simulink model "bolide_modele_simul2"  (R2023b)
settings: Solver=VariableStepAuto  StartTime=0.0  StopTime=5.0  RelTol=1e-3
model workspace (MATLAB code in the model file):
  | %% True Parameters
  | % Masses
  | mw=0.1;
  | mb=1;
  | M=1.2;
  | 
  | % Distances
  | rho=0.07;
  | l=0.02;
  | d=0.015; % distance A-C
  | 
  | % Electriques
  | L=0.05;
  | R=1e6;
  | % r;
  | 
  | % Couples
  | k=2.63e4;
  | % alpha=34.6;
  | % beta=2.06e5;
  | 
  | % Moments inertie
  | Iwy=2.45e-4;
  | Ipsi=1.53e-2;
  | 
  | % Utilitaire
  | beta = (M + 2*Iwy/rho^2);
  | gamma = Ipsi + mb*d^2;
  | 
  | %% Nominal Equilibrium Point
  | Ubar = 12;
  | Urbar = Ubar/2;
  | Ulbar = Ubar/2;
  | 
  | ubar = rho/2/k*Ubar; % m/s
  | psibar = 0;
  | vbar = 0;
  | irbar = 0;
  | ilbar = 0;
  | 
  | statebar = [ubar; psibar; vbar; irbar; ilbar];
settings Model: Creator=Jules  LastModifiedBy=Jules

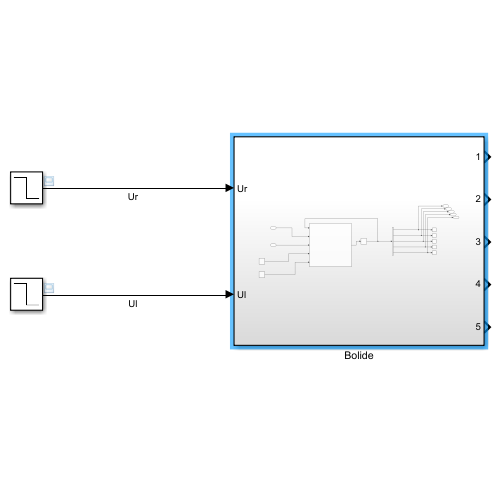
[thumbnail: Simulink's stored preview of the top-level diagram]
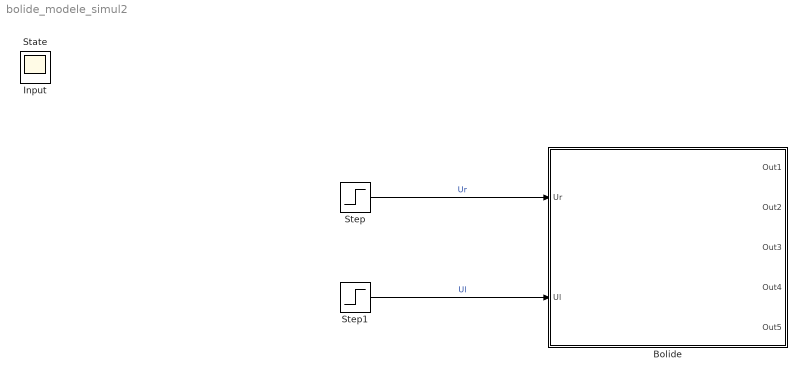
== system bolide_modele_simul2 ==
  Bolide : Subsystem
  Step : Step  Before=Urbar  After=Urbar - 0.1  SampleTime=0
  Step1 : Step  Time=3  Before=Ulbar  After=Ulbar - 0.3  SampleTime=0
  Input : Scope
  State : Scope
  wires:
  Step/1 -> Bolide/1(Ur)  "Ur"
  Step1/1 -> Bolide/2(Ul)  "Ul"

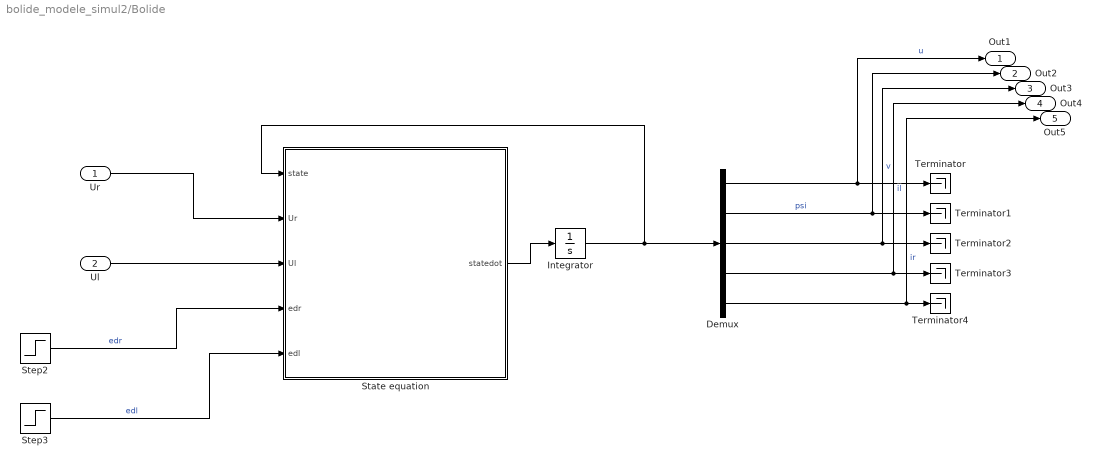
== system bolide_modele_simul2/Bolide ==
  Ur : Inport
  Ul : Inport  Port=2
  Demux : Demux  Outputs=5
  Integrator : Integrator  InitialCondition=statebar
  State equation : MATLAB Function  TreatAsAtomicUnit=on
  Step2 : Step  After=0  SampleTime=0
  Step3 : Step  After=0  SampleTime=0
  Terminator{,1..4} (5 alike) : Terminator
  Out1 : Outport
  Out2 : Outport  Port=2
  Out3 : Outport  Port=3
  Out4 : Outport  Port=4
  Out5 : Outport  Port=5
  wires:
  Step3/1 -> State equation/5(edl)  "edl"
  State equation/1(statedot) -> Integrator/1
  Integrator/1 -> State equation/1(state), Demux/1
  Demux/1 -> Out1/1, Terminator/1  "u"
  Demux/4 -> Out4/1, Terminator3/1  "il"
  Demux/5 -> Out5/1, Terminator4/1  "ir"
  Demux/2 -> Out2/1, Terminator1/1  "psi"
  Demux/3 -> Out3/1, Terminator2/1  "v"
  Step2/1 -> State equation/4(edr)  "edr"
  Ul/1 -> State equation/3(Ul)
  Ur/1 -> State equation/2(Ur)

== matlab function bolide_modele_simul2/Bolide/State equation ==
  data: state input; statedot output; Ur input; Ul input; edr input; edl input; M parameter; rho parameter; l parameter; Iwy parameter; Ipsi parameter; d parameter; L parameter; R parameter; k parameter; mb parameter; beta parameter; gamma parameter
function statedot = fcn(state,Ur, Ul, edr, edl, M, rho, l, Iwy, Ipsi, d, L, R, k, mb, beta, gamma)
% ed est l'entrée de perturbation, != d (distance AC)
% Model parameters M,Ipsi,d,L,R,k defined in "Model Explorer/Matlab Code"

u = state(1);
psi = state(2);
v = state(3); % psidot
ir = state(4); % Intensité à gauche
il = state(5);

is = ir + il; % Somme
id = ir - il; % Diff
Us = Ur + Ul + edr + edl;
Ud = Ur - Ul + edr - edl;

udot = 1/beta*(k/rho*is - mb*d*v^2);
psidot = v;
vdot = 1/gamma*(l*k/(2*rho)*id + mb*d*u*v);
isdot = 1/L*(Us - R*is - 2*k/rho*u);
iddot = 1/L*(Ud - R*id - k*l/rho*v);

irdot = 0.5*(isdot + iddot);
ildot = 0.5*(isdot - iddot);

statedot = [udot; psidot; vdot; irdot; ildot];
